simulink model "simulation_w_switch_sln3"  (Simulink 10.1)
settings: Solver=VariableStepAuto  StartTime=0.0  StopTime=tTot  MaxStep=1e-5  RelTol=1e-5
PreLoadFcn:
  | syst_init
values from neighbouring files (symbols this model uses):
  Aij = Aconn-Aii    [syst_init.m]
  AL = blkdiag(DGU.ALi)    [syst_init.m]
  atk24 = [zeros(3,1); 0.1*rand(3,1)-0.05]    [syst_init.m]
  atk34 = [zeros(3,1); 0.1*rand(3,1)-0.05]    [syst_init.m]
  B = blkdiag(DGU.B)    [syst_init.m]
  bC = blkdiag(DGU.bC)    [syst_init.m]
  bF = blkdiag(DGU.bF)    [syst_init.m]
  bH = blkdiag(DGU.bH)    [syst_init.m]
  bigCyComm = [zeros(3,3)  eye(3) zeros(3,30) ... (first row only)    [syst_init.m]
  bKhat = blkdiag(DGU.bKhat)    [syst_init.m]
  DGU = stateDyn(DGU,6)    [syst_init.m]
  F = blkdiag(DGU.Fj)    [syst_init.m]
  H = blkdiag(DGU.Hj)    [syst_init.m]
  K = blkdiag(DGU.K)    [syst_init.m]
  Khat = blkdiag(DGU.Khat)    [syst_init.m]
  L = blkdiag(DGU.Li)    [syst_init.m]
  n = 3    [syst_init.m]
  N = 6    [syst_init.m]
  nMaxMeas = .01    (= 0.01)    [syst_init.m]
  rhoMax = nMaxMeas*repmat([ones(n-1,1);0],N,1)    [syst_init.m]
  T = blkdiag(DGU.Tj)    [syst_init.m]
  Ta = 8    [syst_init.m]
  Tc = 2    [syst_init.m]
  tSampData = 1e-3    (= 0.001)    [syst_init.m]
  Vs = 60    [syst_init.m]
  wMax = nMax*repmat([ones(n-1,1);0],N,1)+nMaxMeas*repmat([zeros(n-1,1);1],N,1)    [syst_init.m]
undefined symbols (not defined in the file or in its folder): epsilon0bar, integral_Loc, rLoc_bar
libraries: powerlib x136, powerlib_meascontrol x13
(part 1 of 4)
settings Model: Creator=mustafa  LastModifiedBy=mustafa
settings DataIOCC: SaveFormat=Dataset
settings OptimizationCC: LifeSpan=auto
settings DebuggingCC: UnderspecifiedInitializationDetection=Simplified  MergeDetectMultiDrivingBlocksExec=error  UnconnectedInputMsg=none  UnconnectedOutputMsg=none  UnconnectedLineMsg=none  SFUnexpectedBacktrackingDiag=error  SFNoUnconditionalDefaultTransitionDiag=error  SFExecutionAtInitializationDiag=warning
settings HardwareCC: ProdBitPerPointer=64  ProdBitPerSizeT=64  ProdBitPerPtrDiffT=64  ProdLargestAtomicFloat=Float  ProdIntDivRoundTo=Zero  ProdEndianess=LittleEndian  ProdWordSize=64  ProdHWDeviceType=Intel->x86-64 (Windows64)
settings ModelReferenceCC: PropagateSignalLabelsOutOfModel=on
settings SFSimCC: SimUseLocalCustomCode=on
settings RTWCC: RTWUseLocalCustomCode=on
settings CodeAppCC: StateflowObjectComments=off
settings GRTTargetCC: TargetLangStandard=C99 (ISO)  CombineOutputUpdateFcns=on  GRTInterface=off
settings ConfigComp: CovMetricSettings=dwe  CovHtmlReporting=off  CovSaveCumulativeToWorkspaceVar=off  CovSaveSingleToWorkspaceVar=off  CovExternalEMLEnable=on

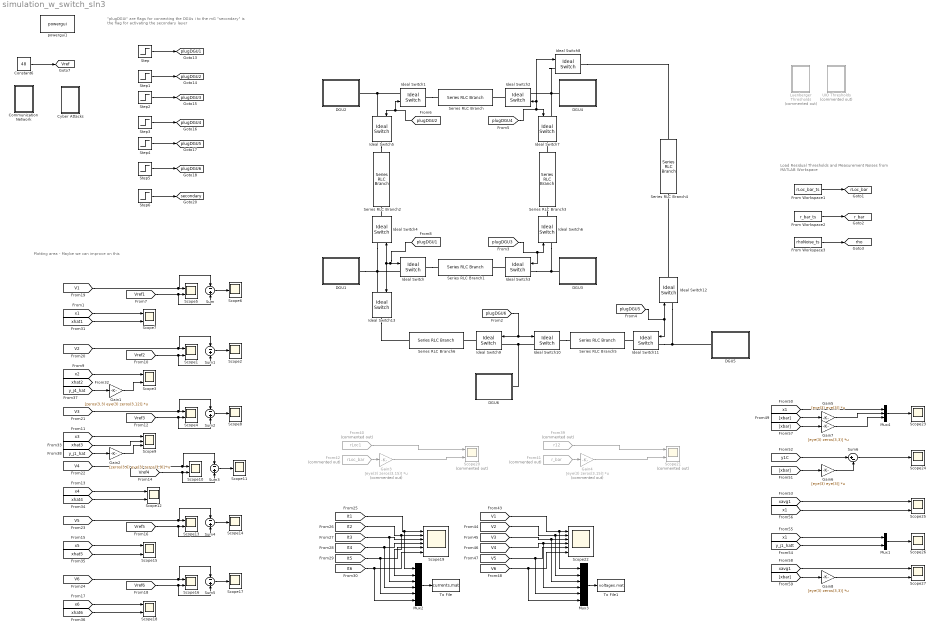
== system simulation_w_switch_sln3 ==
  note: Plotting area - Maybe we can improve on this
  note: "plugDGUi" are flags for connecting the DGUs i to the mG
      | "secondary" is the flag for activating the secondary layer
  note: Load Residual Thresholds and Measurement
      | Noises from MATLAB Workspace
  Communication  Network : Subsystem
  Constant6 : Constant  Value=48
  Cyber Attacks : Subsystem
  DGU1 : Subsystem
  DGU2 : Subsystem
  DGU3 : Subsystem
  DGU4 : Subsystem
  DGU5 : Subsystem
  DGU6 : Subsystem
  From Workspace1 : FromWorkspace  VariableName=rLoc_bar_ts
  From Workspace2 : FromWorkspace  VariableName=r_bar_ts
  From Workspace3 : FromWorkspace  VariableName=rhoNoise_ts
  From39 : From  Commented=on  GotoTag=r12  TagVisibility=global
  From40 : From  Commented=on  GotoTag=rLoc1  TagVisibility=global
  From41 : From  Commented=on  GotoTag=r_bar  TagVisibility=global
  From42 : From  Commented=on  GotoTag=rLoc_bar  TagVisibility=global
  Gain1 : Gain  Gain=[zeros(3,3) eye(3) zeros(3,12)]  Multiplication=Matrix(K*u) (u vector)
  Gain2 : Gain  Gain=[zeros(3,6) eye(3) zeros(3,9)]  Multiplication=Matrix(K*u) (u vector)
  Gain3 : Gain  Commented=on  Gain=[eye(3) zeros(3,15)]  Multiplication=Matrix(K*u) (u vector)
  Gain4 : Gain  Commented=on  Gain=[eye(3) zeros(3,15)]  Multiplication=Matrix(K*u) (u vector)
  Gain5 : Gain  Gain=[eye(3) eye(3)]  Multiplication=Matrix(K*u) (u vector)
  Gain6 : Gain  Gain=[eye(3) eye(3)]  Multiplication=Matrix(K*u) (u vector)
  Gain7 : Gain  Gain=[eye(3) zeros(3,3)]  Multiplication=Matrix(K*u) (u vector)
  Gain8 : Gain  Gain=[eye(3) zeros(3,3)]  Multiplication=Matrix(K*u) (u vector)
  Ideal Switch{,1..13} (14 alike) : powerlib/Power Electronics/Ideal Switch  Ron=0.001  Lon=0  IC=0  Rs=1e5  Cs=inf  Measurements=off
  Luenberger Thresholds : Subsystem  Commented=on
  Mux1 : Mux  Inputs=2
  Mux2 : Mux  Inputs=6
  Mux3 : Mux  Inputs=6
  Mux4 : Mux  Inputs=3
  Scope{1,4..5,7,10,12..13,15..16,18,25,27} (12 alike) : Scope  NumInputPorts=2
  Scope{2,6,8,11,14,17,23..24,26} (9 alike) : Scope
  Scope19 : Scope  NumInputPorts=6
  Scope20 : Scope  Commented=on  NumInputPorts=2
  Scope21 : Scope  Commented=on  NumInputPorts=2
  Scope22 : Scope  NumInputPorts=6
  Scope3 : Scope  NumInputPorts=3
  Scope9 : Scope  NumInputPorts=3
  Series RLC Branch : powerlib/Elements/Series RLC Branch  LConnTagsString=__new0  RConnTagsString=__new0  BranchType=RL  Resistance=DGU(2).Rij(2)  Inductance=DGU(2).Lij(2)  SetiL0=off  InitialCurrent=0  Capacitance=1e-6  Setx0=off  InitialVoltage=0  Measurements=None
  Series RLC Branch1 : powerlib/Elements/Series RLC Branch  LConnTagsString=__new0  RConnTagsString=__new0  BranchType=RL  Resistance=DGU(1).Rij(2)  Inductance=DGU(1).Lij(2)  SetiL0=off  InitialCurrent=0  Capacitance=1e-6  Setx0=off  InitialVoltage=0  Measurements=None
  Series RLC Branch2 : powerlib/Elements/Series RLC Branch  LConnTagsString=__new0  RConnTagsString=__new0  BranchType=RL  Resistance=DGU(1).Rij(1)  Inductance=DGU(1).Lij(1)  SetiL0=off  InitialCurrent=0  Capacitance=1e-6  Setx0=off  InitialVoltage=0  Measurements=None
  Series RLC Branch3 : powerlib/Elements/Series RLC Branch  LConnTagsString=__new0  RConnTagsString=__new0  BranchType=RL  Resistance=DGU(3).Rij(2)  Inductance=DGU(3).Lij(2)  SetiL0=off  InitialCurrent=0  Capacitance=1e-6  Setx0=off  InitialVoltage=0  Measurements=None
  Series RLC Branch4 : powerlib/Elements/Series RLC Branch  LConnTagsString=__new0  RConnTagsString=__new0  BranchType=RL  Resistance=DGU(4).Rij(3)  Inductance=DGU(4).Lij(3)  SetiL0=off  InitialCurrent=0  Capacitance=1e-6  Setx0=off  InitialVoltage=0  Measurements=None
  Series RLC Branch5 : powerlib/Elements/Series RLC Branch  LConnTagsString=__new0  RConnTagsString=__new0  BranchType=RL  Resistance=DGU(5).Rij(2)  Inductance=DGU(5).Lij(2)  SetiL0=off  InitialCurrent=0  Capacitance=1e-6  Setx0=off  InitialVoltage=0  Measurements=None
  Series RLC Branch6 : powerlib/Elements/Series RLC Branch  LConnTagsString=__new0  RConnTagsString=__new0  BranchType=RL  Resistance=DGU(1).Rij(3)  Inductance=DGU(1).Lij(3)  SetiL0=off  InitialCurrent=0  Capacitance=1e-6  Setx0=off  InitialVoltage=0  Measurements=None
  Step{,1..6} (7 alike) : Step  Time=Tc  SampleTime=0
  Sum{,1..5} (6 alike) : Sum  Inputs=-|+
  Sum6 : Sum  Inputs=|+-
  To File : ToFile  Filename=currents.mat  MatrixName=currents  SaveFormat=Timeseries  SampleTime=tSampData
  To File1 : ToFile  Filename=voltages.mat  MatrixName=voltages  SaveFormat=Timeseries  SampleTime=tSampData
  UIO Thresholds : Subsystem  Commented=on
  powergui1 : powerlib/powergui  Priority=1  SimulationMode=Continuous  SampleTime=50e-6  frequency=60  Iterations=50  frequencyindice=0  Pbase=100e6  ErrMax=1e-4  UnitsV=kV  UnitsW=MW  buscounter=0  FunctionMessages=off  echomessages=off  EnableUseOfTLC=off  CurrentSourceSwitches=off  DisableSnubberDevices=off  DisableRonSwitches=off  DisableVfSwitches=off  DisplayEquations=off  AutomaticDiscreteSolvers=off  SolverType=Tustin/Backward Euler (TBE)  Interpol=off  ExternalGateDelay=off  methode=off  Ts=100  x0status=blocks  SPID=on  SwTol=0  HookPort=off  NonlinearTolerance=1e-4  nMaxIteration=100  ContinueOnMaxIteration=off  RestoreLinks=warning  ResistiveCurrentMeasurement=off  Frange=[0:2:500]  Ylog=off  Xlog=on  ShowGrid=off  save=off  variable=ZData  structure=0  ZoomFFT=off  StartTime=0.0  cycles=1  DisplayStyle=1  fundamental=60  FreqAxis=off  MaxFrequency=1000  frequencyindicesteady=1  RmsSteady=1  display=off
  tag scope: Vref=global, plugDGU1=global, plugDGU2=global, plugDGU3=global, plugDGU4=global, plugDGU5=global, plugDGU6=global, rLoc_bar=global, r_bar=global, rho=global, secondary=global
  wires:
  [Vref1] -> Sum/2, Scope5/2
  [V1] -> Sum/1, Scope5/1
  Sum/1 -> Scope6/1
  [x1] -> Scope7/1
  [plugDGU2] -> Ideal Switch1/1, Ideal Switch5/1
  [plugDGU1] -> Ideal Switch4/1, Ideal Switch13/1, Ideal Switch/1
  [plugDGU3] -> Ideal Switch6/1, Ideal Switch3/1
  [plugDGU4] -> Ideal Switch7/1, Ideal Switch8/1, Ideal Switch2/1
  [plugDGU6] -> Ideal Switch9/1, Ideal Switch10/1
  [plugDGU5] -> Ideal Switch11/1, Ideal Switch12/1
  [V2] -> Sum1/1, Scope1/1
  [Vref2] -> Sum1/2, Scope1/2
  Sum1/1 -> Scope2/1
  [x2] -> Scope3/1
  [V3] -> Sum2/1, Scope4/1
  [Vref3] -> Sum2/2, Scope4/2
  Sum2/1 -> Scope8/1
  [x3] -> Scope9/1
  [V4] -> Sum3/1, Scope10/1
  [Vref4] -> Sum3/2, Scope10/2
  Sum3/1 -> Scope11/1
  [x4] -> Scope12/1
  [V5] -> Sum4/1, Scope13/1
  [Vref5] -> Sum4/2, Scope13/2
  Sum4/1 -> Scope14/1
  [x5] -> Scope15/1
  [V6] -> Sum5/1, Scope16/1
  [Vref6] -> Sum5/2, Scope16/2
  Sum5/1 -> Scope17/1
  [x6] -> Scope18/1
  Step/1 -> [plugDGU1]
  Step1/1 -> [plugDGU2]
  Step2/1 -> [plugDGU3]
  Step3/1 -> [plugDGU4]
  Step4/1 -> [plugDGU5]
  Step5/1 -> [plugDGU6]
  Constant6/1 -> [Vref]
  Step6/1 -> [secondary]
  [It3] -> Mux2/3, Scope19/3
  [It2] -> Mux2/2, Scope19/2
  [It1] -> Mux2/1, Scope19/1
  [It4] -> Mux2/4, Scope19/4
  [It5] -> Mux2/5, Scope19/5
  [It6] -> Mux2/6, Scope19/6
  [xhat1] -> Scope7/2
  [xhat3] -> Scope9/2
  [xhat4] -> Scope12/2
  [xhat5] -> Scope15/2
  [xhat6] -> Scope18/2
  [y_j4_hat] -> Gain1/1
  Gain1/1 -> Scope3/3
  [y_j1_hat] -> Gain2/1
  Gain2/1 -> Scope9/3
  From42/1 -> Gain3/1
  From41/1 -> Gain4/1
  From40/1 -> Scope20/1
  Gain4/1 -> Scope21/2
  Gain3/1 -> Scope20/2
  From39/1 -> Scope21/1
  [V6] -> Mux3/6, Scope22/6
  [V1] -> Mux3/1, Scope22/1
  [V4] -> Scope22/4, Mux3/4
  [V3] -> Mux3/3, Scope22/3
  [V2] -> Mux3/2, Scope22/2
  [V5] -> Mux3/5, Scope22/5
  Mux4/1 -> Scope23/1
  [x1] -> Mux4/1
  Sum6/1 -> Scope24/1
  Gain5/1 -> Mux4/2
  [xbar] -> Gain6/1
  Gain6/1 -> Sum6/2
  [xbar] -> Gain5/1
  [y1C] -> Sum6/1
  [xavg1] -> Scope25/1
  [y_j1_hatt] -> Mux1/2
  [x1] -> Mux1/1
  Mux1/1 -> Scope26/1
  [x1] -> Scope25/2
  [xbar] -> Gain7/1
  Gain7/1 -> Mux4/3
  [xavg1] -> Scope27/1
  [xbar] -> Gain8/1
  Gain8/1 -> Scope27/2
  From Workspace1/1 -> [rLoc_bar]
  From Workspace2/1 -> [r_bar]
  From Workspace3/1 -> [rho]
  Mux2/1 -> To File/1
  Mux3/1 -> To File1/1
  connections:
  Ideal Switch/RConn1 -- Series RLC Branch1/LConn1
  Ideal Switch1/RConn1 -- Series RLC Branch/LConn1
  Ideal Switch4/RConn1 -- Series RLC Branch2/RConn1
  DGU1/RConn1 -- Ideal Switch13/LConn1 -- Ideal Switch4/LConn1 -- Ideal Switch/LConn1
  Ideal Switch5/RConn1 -- Series RLC Branch2/LConn1
  Ideal Switch1/LConn1 -- Ideal Switch5/LConn1 -- DGU2/RConn1
  Ideal Switch3/RConn1 -- Series RLC Branch1/RConn1
  Ideal Switch2/RConn1 -- Series RLC Branch/RConn1
  Ideal Switch3/LConn1 -- Ideal Switch6/LConn1 -- DGU3/LConn1
  Ideal Switch2/LConn1 -- Ideal Switch8/LConn1 -- Ideal Switch7/LConn1 -- DGU4/LConn1
  Series RLC Branch3/LConn1 -- Ideal Switch7/RConn1
  Series RLC Branch3/RConn1 -- Ideal Switch6/RConn1
  Ideal Switch8/RConn1 -- Series RLC Branch4/LConn1
  Ideal Switch9/RConn1 -- Series RLC Branch6/RConn1
  Ideal Switch10/RConn1 -- Series RLC Branch5/LConn1
  Ideal Switch10/LConn1 -- Ideal Switch9/LConn1 -- DGU6/RConn1
  Ideal Switch11/RConn1 -- Series RLC Branch5/RConn1
  Ideal Switch11/LConn1 -- Ideal Switch12/LConn1 -- DGU5/LConn1
  Ideal Switch13/RConn1 -- Series RLC Branch6/LConn1
  Ideal Switch12/RConn1 -- Series RLC Branch4/RConn1

== system simulation_w_switch_sln3/Communication  Network ==
  Constant : Constant  Value=zeros(2*n*N,1)
  Gain : Gain  Gain=blkdiag(zeros(6),eye(6),eye(6),zeros(6),zeros(6),eye(6))  Multiplication=Matrix(K*u) (u vector)
  Gain1 : Gain  Gain=blkdiag(eye(6),zeros(6),zeros(6),eye(6),zeros(6),zeros(6))  Multiplication=Matrix(K*u) (u vector)
  Gain2 : Gain  Gain=blkdiag(eye(6),zeros(6),zeros(6),eye(6),zeros(6),zeros(6))  Multiplication=Matrix(K*u) (u vector)
  Gain3 : Gain  Gain=blkdiag(zeros(6),eye(6),eye(6),zeros(6),eye(6),zeros(6))  Multiplication=Matrix(K*u) (u vector)
  Gain4 : Gain  Gain=blkdiag(zeros(6),zeros(6),zeros(6),eye(6),zeros(6),eye(6))  Multiplication=Matrix(K*u) (u vector)
  Gain5 : Gain  Gain=blkdiag(eye(6),zeros(6),zeros(6),zeros(6),eye(6),zeros(6))  Multiplication=Matrix(K*u) (u vector)
  Mux : Mux  Inputs=12
  Switch : Switch  Criteria=u2 > Threshold  Threshold=0.1
  tag scope: yCom1=global, yCom2=global, yCom3=global, yCom4=global, yCom5=global, yCom6=global, yTot=global
  wires:
  [y1] -> Mux/2
  Gain/1 -> [yCom1]
  Gain3/1 -> [yCom4]
  [y6] -> Mux/12
  [y5] -> Mux/10
  [y4] -> Mux/8
  [yTot] -> Gain1/1, Gain2/1, Gain3/1, Gain4/1, Gain5/1, Gain/1
  Gain5/1 -> [yCom6]
  [y3] -> Mux/6
  [y2] -> Mux/4
  Gain4/1 -> [yCom5]
  Gain1/1 -> [yCom2]
  Gain2/1 -> [yCom3]
  Constant/1 -> Switch/3
  [secondary] -> Switch/2
  Switch/1 -> [yTot]
  Mux/1 -> Switch/1
  [xavg6] -> Mux/11
  [xavg1] -> Mux/1
  [xavg2] -> Mux/3
  [xavg3] -> Mux/5
  [xavg4] -> Mux/7
  [xavg5] -> Mux/9

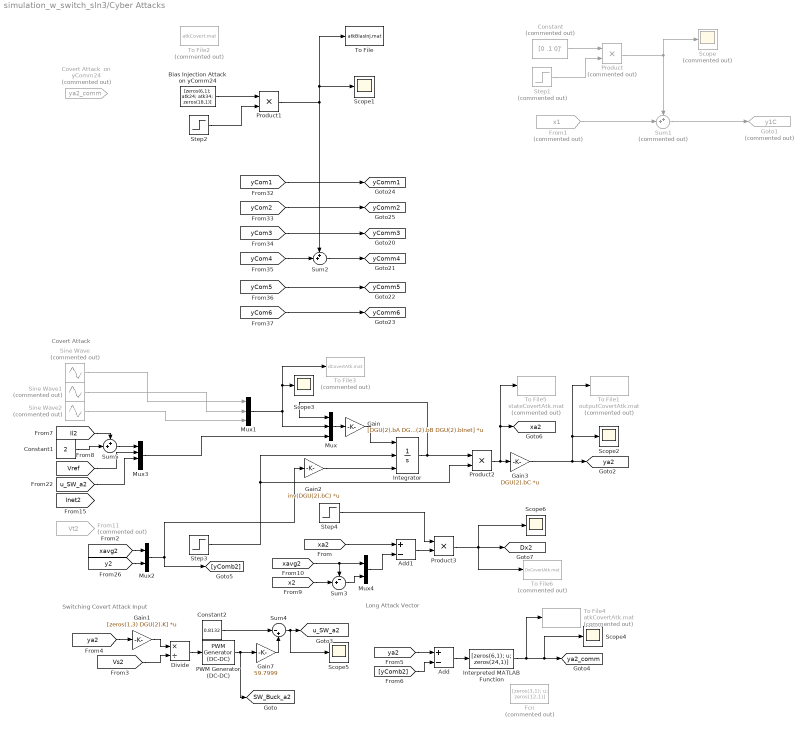
== system simulation_w_switch_sln3/Cyber Attacks ==
  note: Long Attack Vector
  note: Switching Covert Attack Input
  note: Covert Attack
  Add : Sum  Inputs=+-
  Add1 : Sum  Inputs=+-
  Bias Injection Attack on yComm24 : Constant  Value=[zeros(6,1); atk24; atk34; zeros(18,1)]
  Constant : Constant  Commented=on  Value=[0 .1 0]'
  Constant1 : Constant  Value=2
  Constant2 : Constant  Value=0.8132
  Covert Attack  on yComm24 : From  Commented=on  GotoTag=ya2_comm  TagVisibility=global
  Divide : Product  Inputs=*/
  Fcn : Fcn  Commented=on  Expr=[zeros(3,1); u; zeros(12,1)]
  From1 : From  Commented=on  GotoTag=x1  TagVisibility=global
  From11 : From  Commented=on  GotoTag=Vt2  TagVisibility=global
  Gain : Gain  Gain=[DGU(2).bA DGU(2).bEbar DGU(2).bM DGU(2).bB DGU(2).bInet]  Multiplication=Matrix(K*u) (u vector)
  Gain1 : Gain  Gain=[zeros(1,3) DGU(2).K]  Multiplication=Matrix(K*u) (u vector)
  Gain2 : Gain  Gain=inv(DGU(2).bC)  Multiplication=Matrix(K*u) (u vector)
  Gain3 : Gain  Gain=DGU(2).bC  Multiplication=Matrix(K*u) (u vector)
  Gain7 : Gain  Gain=59.7999
  Goto1 : Goto  Commented=on  GotoTag=y1C  TagVisibility=global
  Integrator : Integrator  ExternalReset=rising  InitialConditionSource=external
  Interpreted MATLAB Function : MATLABFcn  MATLABFcn=[zeros(6,1); u; zeros(24,1)]
  Mux : Mux  Inputs=3
  Mux1 : Mux  Inputs=3
  Mux2 : Mux  Inputs=2
  Mux3 : Mux
  Mux4 : Mux  Inputs=2
  PWM Generator (DC-DC) : powerlib_meascontrol/Pulse & Signal Generators/PWM Generator (DC-DC)  Fsw=10000  Ts=0
  Product : Product  Commented=on
  Product1 : Product
  Product2 : Product
  Product3 : Product
  Scope : Scope  Commented=on
  Scope{1..6} (6 alike) : Scope
  Sine Wave : Sin  Commented=on  Amplitude=1.2  Bias=1  Frequency=2*pi*0.1  Phase=90  SampleTime=0
  Sine Wave1 : Sin  Commented=on  Bias=0.5  Frequency=2*pi*0.2  SampleTime=0
  Sine Wave2 : Sin  Commented=on  Amplitude=0.8  Bias=0.6  Frequency=2*pi*0.15  SampleTime=0
  Step1 : Step  Commented=on  Time=8  SampleTime=0
  Step2 : Step  Time=Ta  SampleTime=0
  Step3 : Step  Time=Ta  SampleTime=0
  Step4 : Step  Time=Ta  SampleTime=0
  Sum1 : Sum  Commented=on  Inputs=++|
  Sum2 : Sum  Inputs=++|
  Sum3 : Sum  Inputs=-+|
  Sum4 : Sum  Inputs=|-+
  Sum5 : Sum  Inputs=++|
  To File : ToFile  Filename=atkBiasInj.mat  MatrixName=atkBiasInj  SaveFormat=Timeseries  SampleTime=tSampData
  To File1 : ToFile  Commented=on  Filename=outputCovertAtk.mat  MatrixName=outputCovertAtk  SaveFormat=Timeseries  SampleTime=tSampData
  To File2 : ToFile  Commented=on  Filename=atkCovert.mat  MatrixName=atkCovert  SaveFormat=Timeseries  SampleTime=tSampData
  To File3 : ToFile  Commented=on  Filename=dCovertAtk.mat  MatrixName=dCovertAtk  SaveFormat=Timeseries  SampleTime=tSampData
  To File4 : ToFile  Commented=on  Filename=atkCovertAtk.mat  MatrixName=atkCovertAtk  SaveFormat=Timeseries  SampleTime=tSampData
  To File5 : ToFile  Commented=on  Filename=stateCovertAtk.mat  MatrixName=stateCovertAtk  SaveFormat=Timeseries  SampleTime=tSampData
  To File6 : ToFile  Commented=on  Filename=DxCovertAtk.mat  MatrixName=DxCovertAtk  SaveFormat=Timeseries  SampleTime=tSampData
  tag scope: Dx2=global, SW_Buck_a2=global, u_SW_a2=global, xa2=global, yComm1=global, yComm2=global, yComm3=global, yComm4=global, yComm5=global, yComm6=global, ya2=global, ya2_comm=global
  wires:
  [yCom1] -> [yComm1]
  [yCom2] -> [yComm2]
  [yCom4] -> Sum2/2
  [yCom5] -> [yComm5]
  [yCom6] -> [yComm6]
  [yCom3] -> [yComm3]
  From1/1 -> Sum1/2
  Sum1/1 -> Goto1/1
  Constant/1 -> Product/1
  Product/1 -> Scope/1, Sum1/1
  Step1/1 -> Product/2
  Step2/1 -> Product1/2
  Product1/1 -> Sum2/1, To File/1, Scope1/1
  Bias Injection Attack on yComm24/1 -> Product1/1
  Sum2/1 -> [yComm4]
  Integrator/1 -> Product2/1, Mux/1
  Step3/1 -> Integrator/2, Product2/2
  Gain/1 -> Integrator/1
  [Vs2] -> Divide/2
  Gain1/1 -> Divide/1
  Divide/1 -> PWM Generator (DC-DC)/1
  [ya2] -> Gain1/1
  Gain7/1 -> Sum4/2
  PWM Generator (DC-DC)/1 -> Gain7/1, [SW_Buck_a2]
  Constant2/1 -> Sum4/1
  Sum4/1 -> Scope5/1, [u_SW_a2]
  Mux/1 -> Gain/1
  Mux1/1 -> Scope3/1, To File3/1, Mux/2
  Sine Wave/1 -> Mux1/1
  Sine Wave1/1 -> Mux1/2
  Product2/1 -> To File5/1, [xa2], Gain3/1
  [ya2] -> Add/1
  [yComb2] -> Add/2
  Add/1 -> Interpreted MATLAB Function/1
  Interpreted MATLAB Function/1 -> To File4/1, Scope4/1, [ya2_comm]
  Mux2/1 -> [yComb2], Gain2/1
  Gain2/1 -> Integrator/3
  [xavg2] -> Mux2/1
  [y2] -> Mux2/2
  Sine Wave2/1 -> Mux1/3
  Gain3/1 -> To File1/1, Scope2/1, [ya2]
  [Il2] -> Sum5/1
  [Vref] -> Mux3/2
  [u_SW_a2] -> Mux3/3
  Mux3/1 -> Mux/3
  [xa2] -> Add1/1
  [xavg2] -> Sum3/1, Mux4/1
  Mux4/1 -> Add1/2
  [x2] -> Sum3/2
  Sum3/1 -> Mux4/2
  Constant1/1 -> Sum5/2
  Sum5/1 -> Mux3/1
  Add1/1 -> Product3/2
  Step4/1 -> Product3/1
  Product3/1 -> To File6/1, [Dx2], Scope6/1

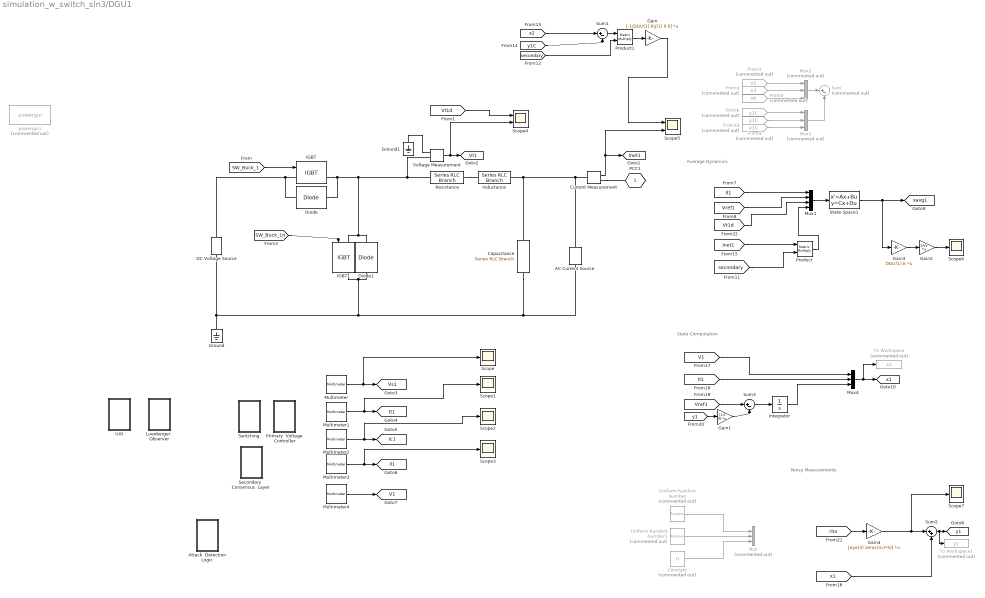
== system simulation_w_switch_sln3/DGU1 ==
  note: Average Dynamics
  note: Noisy Measurements
  note: State Computation
  AC Current Source : powerlib/Electrical Sources/AC Current Source  Amplitude=10  Phase=90  Frequency=0  SampleTime=0  Measurements=Current
      settings: SourceProductBaseCode=PS
  Attack  Detection Logic : Subsystem
  Capacitance : powerlib/Elements/Series RLC Branch  LConnTagsString=__new0  RConnTagsString=__new0  BranchType=C  Resistance=1  Inductance=1.8e-3  SetiL0=off  InitialCurrent=0  Capacitance=DGU(1).Ct  Setx0=off  InitialVoltage=48  Measurements=Branch voltage and current
  Constant : Constant  Commented=on  Value=0
  Current Measurement : powerlib/Measurements/Current Measurement  PhasorSimulation=off  OutputType=Magnitude  PSBequivalent=0
  DC Voltage Source : powerlib/Electrical Sources/DC Voltage Source  Amplitude=Vs  Measurements=Voltage
  Diode : powerlib/Power Electronics/Diode  Ron=0.001  Lon=0  Vf=0.8  IC=0  UseSnubber=0  Rs=500  Cs=250e-9  Measurements=off
  Diode1 : powerlib/Power Electronics/Diode  Ron=0.001  Lon=0  Vf=0.8  IC=0  UseSnubber=0  Rs=500  Cs=250e-9  Measurements=off
  From10 : From  Commented=on  GotoTag=y1C  TagVisibility=global
  From3 : From  Commented=on  GotoTag=x2  TagVisibility=global
  From4 : From  Commented=on  GotoTag=x3  TagVisibility=global
  From5 : From  Commented=on  GotoTag=x6  TagVisibility=global
  From6 : From  Commented=on  GotoTag=y1C  TagVisibility=global
  From9 : From  Commented=on  GotoTag=y1C  TagVisibility=global
  Gain : Gain  Gain=[-1/DGU(1).Rij(1) 0 0]  Multiplication=Matrix(K*u) (u vector)
  Gain1 : Gain  Gain=[1 0 0]  Multiplication=Matrix(K*u) (u vector)
  Gain2 : Gain  Gain=1/Vs  Multiplication=Matrix(K*u) (u vector)
  Gain3 : Gain  Gain=DGU(1).K  Multiplication=Matrix(K*u) (u vector)
  Gain4 : Gain  Gain=[eye(3) zeros(3,n*5)]  Multiplication=Matrix(K*u) (u vector)
  Ground : powerlib/Elements/Ground  LConnTagsString=a
  Ground1 : powerlib/Elements/Ground  LConnTagsString=a
  IGBT : powerlib/Power Electronics/IGBT  Ron=0.001  Lon=0  Vf=1  Tf=1e-6  Tt=2e-6  IC=0  Rs=1e5  Cs=inf  Measurements=on
  IGBT1 : powerlib/Power Electronics/IGBT  Ron=0.001  Lon=0  Vf=1  Tf=1e-6  Tt=2e-6  IC=0  Rs=1e5  Cs=inf  Measurements=on
  Inductance : powerlib/Elements/Series RLC Branch  LConnTagsString=__new0  RConnTagsString=__new0  BranchType=L  Resistance=1  Inductance=DGU(1).Lt  SetiL0=off  InitialCurrent=10  Capacitance=1e-6  Setx0=off  InitialVoltage=0  Measurements=None
  Integrator : Integrator
  Luenberger  Observer : Subsystem
  Multimeter : powerlib/Measurements/Multimeter  PhasorSimulation=off  OutputType=Complex  sel=7  L=30  Gain=1  yselected={'Usrc: DGU1/DC Voltage Source'};  PSBOutputType=1  PSBequivalent=0  AxesSetting=[0,0.1,-100,100]  Display=0  SavedBlockNames=-11
  Multimeter1 : powerlib/Measurements/Multimeter  PhasorSimulation=off  OutputType=Complex  sel=22  L=30  Gain=1  yselected={'Ib: DGU1/Resistance'};  PSBOutputType=1  PSBequivalent=0  AxesSetting=[0,0.1,-100,100]  Display=0  SavedBlockNames=-11
  Multimeter2 : powerlib/Measurements/Multimeter  PhasorSimulation=off  OutputType=Complex  sel=21  L=30  Gain=1  yselected={'Ib: DGU1/Capacitance'};  PSBOutputType=1  PSBequivalent=0  AxesSetting=[0,0.1,-100,100]  Display=0  SavedBlockNames=-11
  Multimeter3 : powerlib/Measurements/Multimeter  PhasorSimulation=off  OutputType=Complex  sel=25  L=30  Gain=1  yselected={'Isrc: DGU1/AC Current Source'};  PSBOutputType=1  PSBequivalent=0  AxesSetting=[0,0.1,-100,100]  Display=0  SavedBlockNames=-11
  Multimeter4 : powerlib/Measurements/Multimeter  PhasorSimulation=off  OutputType=Complex  sel=5  L=30  Gain=1  yselected={'Ub: DGU1/Capacitance'};  PSBOutputType=1  PSBequivalent=0  AxesSetting=[0,0.1,-100,100]  Display=0  SavedBlockNames=-11
  Mux : Mux  Commented=on  Inputs=3
  Mux1 : Mux
  Mux2 : Mux  Commented=on  Inputs=3
  Mux3 : Mux  Commented=on  Inputs=3
  Mux4 : Mux  Inputs=3
  Primary  Voltage  Controller : Subsystem
  Product : Product  Multiplication=Matrix(*)
  Product1 : Product  Multiplication=Matrix(*)
  Resistance : powerlib/Elements/Series RLC Branch  LConnTagsString=__new0  RConnTagsString=__new0  BranchType=R  Resistance=DGU(1).Rt  Inductance=1e-3  SetiL0=off  InitialCurrent=0  Capacitance=1e-6  Setx0=off  InitialVoltage=0  Measurements=Branch current
  Scope{,1..3,6..7} (6 alike) : Scope
  Scope4 : Scope  NumInputPorts=2
  Scope5 : Scope  NumInputPorts=2
  Secondary  Consensus  Layer : Subsystem
  State-Space1 : StateSpace  A=DGU(1).Aii  B=[DGU(1).M DGU(1).B [-1/DGU(1).Ct;0;0]]  C=eye(3)  D=zeros(n,4)  InitialCondition=0
  Sum : Sum  Commented=on  Inputs=|+-
  Sum1 : Sum  Inputs=|+-
  Sum2 : Sum  Inputs=|++
  Sum3 : Sum  Inputs=|+-
  Switching : Subsystem
  To Workspace : ToWorkspace  Commented=on  VariableName=x1  SaveFormat=Timeseries  SampleTime=tSampData
  To Workspace1 : ToWorkspace  Commented=on  VariableName=y1  SaveFormat=Timeseries  SampleTime=tSampData
  UIO : Subsystem
  Uniform Random Number : UniformRandomNumber  Commented=on  Minimum=-nMaxMeas  Maximum=nMaxMeas  Seed=1  SampleTime=0.1
  Uniform Random Number1 : UniformRandomNumber  Commented=on  Minimum=-nMaxMeas  Maximum=nMaxMeas  Seed=2  SampleTime=0.1
  Voltage Measurement : powerlib/Measurements/Voltage Measurement  PhasorSimulation=off  OutputType=Complex  PSBequivalent=0
  powergui1 : powerlib/powergui  Priority=1  Commented=on  SimulationMode=Continuous  SampleTime=50e-6  frequency=60  Iterations=50  frequencyindice=60  Pbase=100e6  ErrMax=1e-4  UnitsV=kV  UnitsW=MW  buscounter=0  FunctionMessages=off  echomessages=off  EnableUseOfTLC=off  CurrentSourceSwitches=off  DisableSnubberDevices=off  DisableRonSwitches=off  DisableVfSwitches=off  DisplayEquations=off  AutomaticDiscreteSolvers=off  SolverType=Tustin/Backward Euler (TBE)  Interpol=off  ExternalGateDelay=off  methode=off  Ts=100  x0status=blocks  SPID=on  SwTol=0  HookPort=off  NonlinearTolerance=1e-4  nMaxIteration=100  ContinueOnMaxIteration=off  RestoreLinks=warning  ResistiveCurrentMeasurement=off  Frange=[0:2:500]  Ylog=off  Xlog=on  ShowGrid=off  save=off  variable=ZData  structure=0  ZoomFFT=off  StartTime=0.0  cycles=1  DisplayStyle=1  fundamental=60  FreqAxis=off  MaxFrequency=1000  frequencyindicesteady=1  RmsSteady=1  display=off
  PCC1 : PMIOPort  Tag=PMCPort  Side=Right
  tag scope: Ic1=global, Il1=global, Inet1=global, It1=global, V1=global, Vs1=global, Vt1=global, x1=global, xavg1=global, y1=global
  wires:
  Multimeter/1 -> Scope/1, [Vs1]
  Multimeter2/1 -> Scope2/1, [Ic1]
  Voltage Measurement/1 -> Scope4/2, [Vt1]
  Multimeter1/1 -> Scope1/1, [It1]
  [SW_Buck_1n] -> IGBT1/1
  Multimeter3/1 -> Scope3/1, [Il1]
  [SW_Buck_1] -> IGBT/1
  Multimeter4/1 -> [V1]
  [Vt1d] -> Scope4/1
  [Il1] -> Mux1/1
  [Vref1] -> Mux1/2
  Gain2/1 -> Scope6/1
  Mux1/1 -> State-Space1/1
  State-Space1/1 -> Gain3/1, [xavg1]
  Gain3/1 -> Gain2/1
  From3/1 -> Mux2/1
  From5/1 -> Mux2/3
  From4/1 -> Mux2/2
  From9/1 -> Mux3/2
  From10/1 -> Mux3/3
  From6/1 -> Mux3/1
  Mux2/1 -> Sum/1
  Mux3/1 -> Sum/2
  [Inet1] -> Product/1
  Product/1 -> Mux1/4
  [secondary] -> Product/2
  Current Measurement/1 -> [Inet1], Scope5/2
  Gain/1 -> Scope5/1
  [y1C] -> Sum1/2
  Product1/1 -> Gain/1
  Sum1/1 -> Product1/1
  [x2] -> Sum1/1
  [secondary] -> Product1/2
  [rho] -> Gain4/1
  [Vref1] -> Sum3/1
  [x1] -> Sum2/2
  Uniform Random Number/1 -> Mux/1
  Sum2/1 -> To Workspace1/1, [y1]
  [It1] -> Mux4/2
  Uniform Random Number1/1 -> Mux/2
  Constant/1 -> Mux/3
  [V1] -> Mux4/1
  Integrator/1 -> Mux4/3
  Sum3/1 -> Integrator/1
  [y1] -> Gain1/1
  Gain1/1 -> Sum3/2
  Gain4/1 -> Sum2/1, Scope7/1
  Mux4/1 -> To Workspace/1, [x1]
  [Vt1d] -> Mux1/3
  connections:
  Ground1/LConn1 -- Voltage Measurement/LConn2
  IGBT1/RConn1 -- AC Current Source/RConn1 -- Capacitance/RConn1 -- Ground/LConn1 -- DC Voltage Source/LConn1 -- Diode1/LConn1
  Capacitance/LConn1 -- Current Measurement/LConn1 -- AC Current Source/LConn1 -- Inductance/RConn1
  IGBT1/LConn1 -- Resistance/LConn1 -- Voltage Measurement/LConn1 -- IGBT/RConn1 -- Diode/LConn1 -- Diode1/RConn1
  IGBT/LConn1 -- Diode/RConn1 -- DC Voltage Source/RConn1
  Resistance/RConn1 -- Inductance/LConn1
  Current Measurement/RConn1 -- PCC1/RConn1

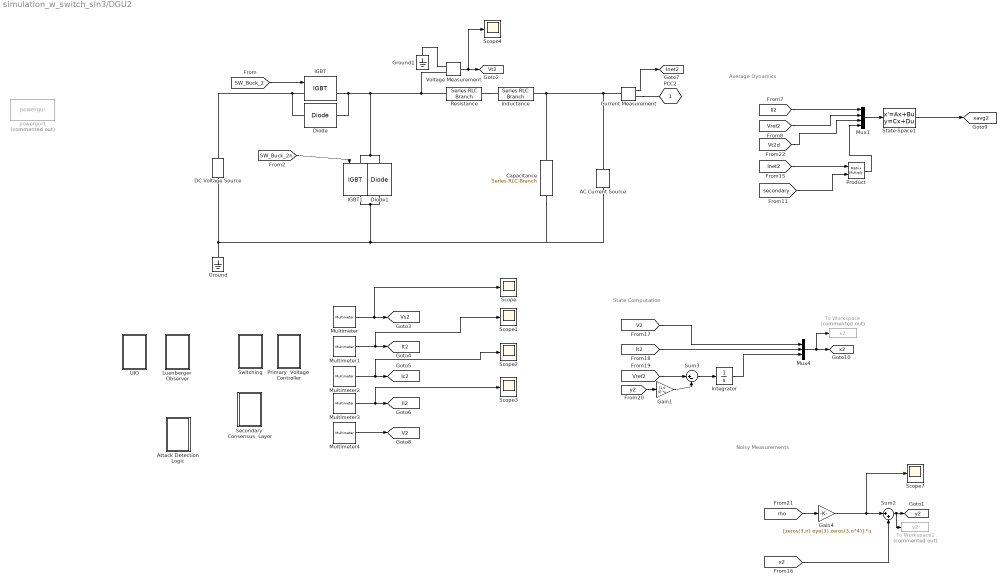
== system simulation_w_switch_sln3/DGU2 ==
  note: Noisy Measurements
  note: State Computation
  note: Average Dynamics
  AC Current Source : powerlib/Electrical Sources/AC Current Source  Amplitude=12  Phase=90  Frequency=0  SampleTime=0  Measurements=Current
      settings: SourceProductBaseCode=PS
  Attack Detection Logic : Subsystem
  Capacitance : powerlib/Elements/Series RLC Branch  LConnTagsString=__new0  RConnTagsString=__new0  BranchType=C  Resistance=1  Inductance=1.8e-3  SetiL0=off  InitialCurrent=0  Capacitance=DGU(2).Ct  Setx0=off  InitialVoltage=48  Measurements=Branch voltage and current
  Current Measurement : powerlib/Measurements/Current Measurement  PhasorSimulation=off  OutputType=Magnitude  PSBequivalent=0
  DC Voltage Source : powerlib/Electrical Sources/DC Voltage Source  Amplitude=Vs  Measurements=Voltage
  Diode : powerlib/Power Electronics/Diode  Ron=0.001  Lon=0  Vf=0.8  IC=0  UseSnubber=0  Rs=500  Cs=250e-9  Measurements=off
  Diode1 : powerlib/Power Electronics/Diode  Ron=0.001  Lon=0  Vf=0.8  IC=0  UseSnubber=0  Rs=500  Cs=250e-9  Measurements=off
  Gain1 : Gain  Gain=[1 0 0]  Multiplication=Matrix(K*u) (u vector)
  Gain4 : Gain  Gain=[zeros(3,n) eye(3) zeros(3,n*4)]  Multiplication=Matrix(K*u) (u vector)
  Ground : powerlib/Elements/Ground  LConnTagsString=a
  Ground1 : powerlib/Elements/Ground  LConnTagsString=a
  IGBT : powerlib/Power Electronics/IGBT  Ron=0.001  Lon=0  Vf=1  Tf=1e-6  Tt=2e-6  IC=0  Rs=1e5  Cs=inf  Measurements=on
  IGBT1 : powerlib/Power Electronics/IGBT  Ron=0.001  Lon=0  Vf=1  Tf=1e-6  Tt=2e-6  IC=0  Rs=1e5  Cs=inf  Measurements=on
  Inductance : powerlib/Elements/Series RLC Branch  LConnTagsString=__new0  RConnTagsString=__new0  BranchType=L  Resistance=1  Inductance=DGU(2).Lt  SetiL0=off  InitialCurrent=12  Capacitance=1e-6  Setx0=off  InitialVoltage=0  Measurements=None
  Integrator : Integrator
  Luenberger  Observer : Subsystem
  Multimeter : powerlib/Measurements/Multimeter  PhasorSimulation=off  OutputType=Complex  sel=8  L=30  Gain=1  yselected={'Usrc: DGU2/DC Voltage Source'};  PSBOutputType=1  PSBequivalent=0  AxesSetting=[0,0.1,-100,100]  Display=0  SavedBlockNames=-11
  Multimeter1 : powerlib/Measurements/Multimeter  PhasorSimulation=off  OutputType=Complex  sel=24  L=30  Gain=1  yselected={'Ib: DGU2/Resistance'};  PSBOutputType=1  PSBequivalent=0  AxesSetting=[0,0.1,-100,100]  Display=0  SavedBlockNames=-11
  Multimeter2 : powerlib/Measurements/Multimeter  PhasorSimulation=off  OutputType=Complex  sel=23  L=30  Gain=1  yselected={'Ib: DGU2/Capacitance'};  PSBOutputType=1  PSBequivalent=0  AxesSetting=[0,0.1,-100,100]  Display=0  SavedBlockNames=-11
  Multimeter3 : powerlib/Measurements/Multimeter  PhasorSimulation=off  OutputType=Complex  sel=26  L=30  Gain=1  yselected={'Isrc: DGU2/AC Current Source'};  PSBOutputType=1  PSBequivalent=0  AxesSetting=[0,0.1,-100,100]  Display=0  SavedBlockNames=-11
  Multimeter4 : powerlib/Measurements/Multimeter  PhasorSimulation=off  OutputType=Complex  sel=6  L=30  Gain=1  yselected={'Ub: DGU2/Capacitance'};  PSBOutputType=1  PSBequivalent=0  AxesSetting=[0,0.1,-100,100]  Display=0  SavedBlockNames=-11
  Mux1 : Mux
  Mux4 : Mux  Inputs=3
  Primary  Voltage  Controller : Subsystem
  Product : Product  Multiplication=Matrix(*)
  Resistance : powerlib/Elements/Series RLC Branch  LConnTagsString=__new0  RConnTagsString=__new0  BranchType=R  Resistance=DGU(2).Rt  Inductance=1e-3  SetiL0=off  InitialCurrent=0  Capacitance=1e-6  Setx0=off  InitialVoltage=0  Measurements=Branch current
  Scope{,1..4,7} (6 alike) : Scope
  Secondary  Consensus  Layer : Subsystem
  State-Space1 : StateSpace  A=DGU(2).Aii  B=[DGU(2).M DGU(2).B [-1/DGU(2).Ct;0;0]]  C=eye(3)  D=zeros(n,4)  InitialCondition=0
  Sum2 : Sum  Inputs=|++
  Sum3 : Sum  Inputs=|+-
  Switching : Subsystem
  To Workspace : ToWorkspace  Commented=on  VariableName=x2  SaveFormat=Timeseries  SampleTime=tSampData
  To Workspace1 : ToWorkspace  Commented=on  VariableName=y2  SaveFormat=Timeseries  SampleTime=tSampData
  UIO : Subsystem
  Voltage Measurement : powerlib/Measurements/Voltage Measurement  PhasorSimulation=off  OutputType=Complex  PSBequivalent=0
  powergui1 : powerlib/powergui  Priority=1  Commented=on  SimulationMode=Continuous  SampleTime=50e-6  frequency=60  Iterations=50  frequencyindice=60  Pbase=100e6  ErrMax=1e-4  UnitsV=kV  UnitsW=MW  buscounter=0  FunctionMessages=off  echomessages=off  EnableUseOfTLC=off  CurrentSourceSwitches=off  DisableSnubberDevices=off  DisableRonSwitches=off  DisableVfSwitches=off  DisplayEquations=off  AutomaticDiscreteSolvers=off  SolverType=Tustin/Backward Euler (TBE)  Interpol=off  ExternalGateDelay=off  methode=off  Ts=100  x0status=blocks  SPID=on  SwTol=0  HookPort=off  NonlinearTolerance=1e-4  nMaxIteration=100  ContinueOnMaxIteration=off  RestoreLinks=warning  ResistiveCurrentMeasurement=off  Frange=[0:2:500]  Ylog=off  Xlog=on  ShowGrid=off  save=off  variable=ZData  structure=0  ZoomFFT=off  StartTime=0.0  cycles=1  DisplayStyle=1  fundamental=60  FreqAxis=off  MaxFrequency=1000  frequencyindicesteady=1  RmsSteady=1  display=off
  PCC2 : PMIOPort  Tag=PMCPort  Side=Right
  tag scope: Ic2=global, Il2=global, Inet2=global, It2=global, V2=global, Vs2=global, Vt2=global, x2=global, xavg2=global, y2=global
  wires:
  Multimeter/1 -> Scope/1, [Vs2]
  Multimeter2/1 -> Scope2/1, [Ic2]
  Voltage Measurement/1 -> Scope4/1, [Vt2]
  Multimeter1/1 -> Scope1/1, [It2]
  [SW_Buck_2n] -> IGBT1/1
  Multimeter3/1 -> Scope3/1, [Il2]
  [SW_Buck_2] -> IGBT/1
  Multimeter4/1 -> [V2]
  [rho] -> Gain4/1
  Gain1/1 -> Sum3/2
  [V2] -> Mux4/1
  [Vref2] -> Sum3/1
  [y2] -> Gain1/1
  [It2] -> Mux4/2
  Gain4/1 -> Sum2/1, Scope7/1
  Integrator/1 -> Mux4/3
  Sum3/1 -> Integrator/1
  Sum2/1 -> To Workspace1/1, [y2]
  Mux4/1 -> To Workspace/1, [x2]
  [x2] -> Sum2/2
  [Il2] -> Mux1/1
  Current Measurement/1 -> [Inet2]
  Mux1/1 -> State-Space1/1
  Product/1 -> Mux1/4
  [Inet2] -> Product/1
  [Vref2] -> Mux1/2
  [secondary] -> Product/2
  [Vt2d] -> Mux1/3
  State-Space1/1 -> [xavg2]
  connections:
  Ground1/LConn1 -- Voltage Measurement/LConn2
  IGBT1/RConn1 -- AC Current Source/RConn1 -- Capacitance/RConn1 -- Ground/LConn1 -- DC Voltage Source/LConn1 -- Diode1/LConn1
  Capacitance/LConn1 -- Current Measurement/LConn1 -- AC Current Source/LConn1 -- Inductance/RConn1
  Diode/LConn1 -- IGBT/RConn1 -- Resistance/LConn1 -- Voltage Measurement/LConn1 -- IGBT1/LConn1 -- Diode1/RConn1
  IGBT/LConn1 -- Diode/RConn1 -- DC Voltage Source/RConn1
  Resistance/RConn1 -- Inductance/LConn1
  Current Measurement/RConn1 -- PCC2/RConn1

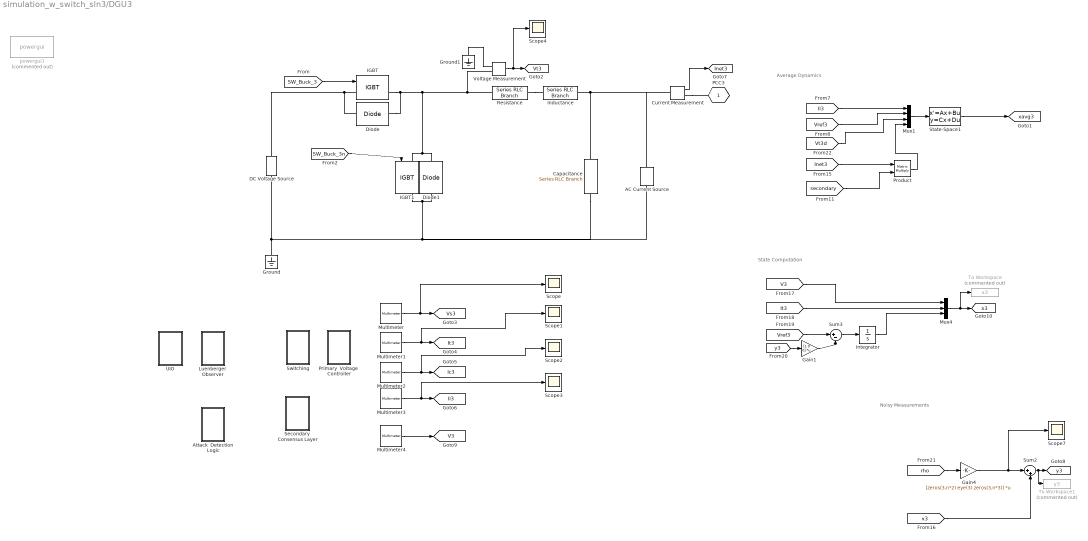
== system simulation_w_switch_sln3/DGU3 ==
  note: Noisy Measurements
  note: State Computation
  note: Average Dynamics
  AC Current Source : powerlib/Electrical Sources/AC Current Source  Amplitude=15  Phase=90  Frequency=0  SampleTime=0  Measurements=Current
      settings: SourceProductBaseCode=PS
  Attack  Detection Logic : Subsystem
  Capacitance : powerlib/Elements/Series RLC Branch  LConnTagsString=__new0  RConnTagsString=__new0  BranchType=C  Resistance=1  Inductance=1.8e-3  SetiL0=off  InitialCurrent=0  Capacitance=DGU(3).Ct  Setx0=off  InitialVoltage=48  Measurements=Branch voltage and current
  Current Measurement : powerlib/Measurements/Current Measurement  PhasorSimulation=off  OutputType=Magnitude  PSBequivalent=0
  DC Voltage Source : powerlib/Electrical Sources/DC Voltage Source  Amplitude=Vs  Measurements=Voltage
  Diode : powerlib/Power Electronics/Diode  Ron=0.001  Lon=0  Vf=0.8  IC=0  UseSnubber=0  Rs=500  Cs=250e-9  Measurements=off
  Diode1 : powerlib/Power Electronics/Diode  Ron=0.001  Lon=0  Vf=0.8  IC=0  UseSnubber=0  Rs=500  Cs=250e-9  Measurements=off
  Gain1 : Gain  Gain=[1 0 0]  Multiplication=Matrix(K*u) (u vector)
  Gain4 : Gain  Gain=[zeros(3,n*2) eye(3) zeros(3,n*3)]  Multiplication=Matrix(K*u) (u vector)
  Ground : powerlib/Elements/Ground  LConnTagsString=a
  Ground1 : powerlib/Elements/Ground  LConnTagsString=a
  IGBT : powerlib/Power Electronics/IGBT  Ron=0.001  Lon=0  Vf=1  Tf=1e-6  Tt=2e-6  IC=0  Rs=1e5  Cs=inf  Measurements=on
  IGBT1 : powerlib/Power Electronics/IGBT  Ron=0.001  Lon=0  Vf=1  Tf=1e-6  Tt=2e-6  IC=0  Rs=1e5  Cs=inf  Measurements=on
  Inductance : powerlib/Elements/Series RLC Branch  LConnTagsString=__new0  RConnTagsString=__new0  BranchType=L  Resistance=1  Inductance=DGU(3).Lt  SetiL0=off  InitialCurrent=15  Capacitance=1e-6  Setx0=off  InitialVoltage=0  Measurements=None
  Integrator : Integrator
  Luenberger  Observer : Subsystem
  Multimeter : powerlib/Measurements/Multimeter  PhasorSimulation=off  OutputType=Complex  sel=9  L=30  Gain=1  yselected={'Usrc: DGU3/DC Voltage Source'};  PSBOutputType=1  PSBequivalent=0  AxesSetting=[0,0.1,-100,100]  Display=0  SavedBlockNames=-11
  Multimeter1 : powerlib/Measurements/Multimeter  PhasorSimulation=off  OutputType=Complex  sel=14  L=30  Gain=1  yselected={'Ib: DGU3/Resistance'};  PSBOutputType=1  PSBequivalent=0  AxesSetting=[0,0.1,-100,100]  Display=0  SavedBlockNames=-11
  Multimeter2 : powerlib/Measurements/Multimeter  PhasorSimulation=off  OutputType=Complex  sel=13  L=30  Gain=1  yselected={'Ib: DGU3/Capacitance'};  PSBOutputType=1  PSBequivalent=0  AxesSetting=[0,0.1,-100,100]  Display=0  SavedBlockNames=-11
  Multimeter3 : powerlib/Measurements/Multimeter  PhasorSimulation=off  OutputType=Complex  sel=27  L=30  Gain=1  yselected={'Isrc: DGU3/AC Current Source'};  PSBOutputType=1  PSBequivalent=0  AxesSetting=[0,0.1,-100,100]  Display=0  SavedBlockNames=-11
  Multimeter4 : powerlib/Measurements/Multimeter  PhasorSimulation=off  OutputType=Complex  sel=1  L=30  Gain=1  yselected={'Ub: DGU3/Capacitance'};  PSBOutputType=1  PSBequivalent=0  AxesSetting=[0,0.1,-100,100]  Display=0  SavedBlockNames=-11
  Mux1 : Mux
  Mux4 : Mux  Inputs=3
  Primary  Voltage  Controller : Subsystem
  Product : Product  Multiplication=Matrix(*)
  Resistance : powerlib/Elements/Series RLC Branch  LConnTagsString=__new0  RConnTagsString=__new0  BranchType=R  Resistance=DGU(3).Rt  Inductance=1e-3  SetiL0=off  InitialCurrent=0  Capacitance=1e-6  Setx0=off  InitialVoltage=0  Measurements=Branch current
  Scope{,1..4,7} (6 alike) : Scope
  Secondary  Consensus Layer : Subsystem
  State-Space1 : StateSpace  A=DGU(3).Aii  B=[DGU(3).M DGU(3).B [-1/DGU(3).Ct;0;0]]  C=eye(3)  D=zeros(n,4)  InitialCondition=0
  Sum2 : Sum  Inputs=|++
  Sum3 : Sum  Inputs=|+-
  Switching : Subsystem
  To Workspace : ToWorkspace  Commented=on  VariableName=x3  SaveFormat=Timeseries  SampleTime=tSampData
  To Workspace1 : ToWorkspace  Commented=on  VariableName=y3  SaveFormat=Timeseries  SampleTime=tSampData
  UIO : Subsystem
  Voltage Measurement : powerlib/Measurements/Voltage Measurement  PhasorSimulation=off  OutputType=Complex  PSBequivalent=0
  powergui1 : powerlib/powergui  Priority=1  Commented=on  SimulationMode=Continuous  SampleTime=50e-6  frequency=60  Iterations=50  frequencyindice=60  Pbase=100e6  ErrMax=1e-4  UnitsV=kV  UnitsW=MW  buscounter=0  FunctionMessages=off  echomessages=off  EnableUseOfTLC=off  CurrentSourceSwitches=off  DisableSnubberDevices=off  DisableRonSwitches=off  DisableVfSwitches=off  DisplayEquations=off  AutomaticDiscreteSolvers=off  SolverType=Tustin/Backward Euler (TBE)  Interpol=off  ExternalGateDelay=off  methode=off  Ts=100  x0status=blocks  SPID=on  SwTol=0  HookPort=off  NonlinearTolerance=1e-4  nMaxIteration=100  ContinueOnMaxIteration=off  RestoreLinks=warning  ResistiveCurrentMeasurement=off  Frange=[0:2:500]  Ylog=off  Xlog=on  ShowGrid=off  save=off  variable=ZData  structure=0  ZoomFFT=off  StartTime=0.0  cycles=1  DisplayStyle=1  fundamental=60  FreqAxis=off  MaxFrequency=1000  frequencyindicesteady=1  RmsSteady=1  display=off
  PCC3 : PMIOPort  Tag=PMCPort  Side=Left
  tag scope: Ic3=global, Il3=global, Inet3=global, It3=global, V3=global, Vs3=global, Vt3=global, x3=global, xavg3=global, y3=global
  wires:
  Multimeter/1 -> Scope/1, [Vs3]
  Multimeter2/1 -> Scope2/1, [Ic3]
  Voltage Measurement/1 -> Scope4/1, [Vt3]
  Multimeter1/1 -> Scope1/1, [It3]
  [SW_Buck_3n] -> IGBT1/1
  Multimeter3/1 -> Scope3/1, [Il3]
  [SW_Buck_3] -> IGBT/1
  Multimeter4/1 -> [V3]
  [rho] -> Gain4/1
  Gain1/1 -> Sum3/2
  [V3] -> Mux4/1
  [Vref3] -> Sum3/1
  [y3] -> Gain1/1
  [It3] -> Mux4/2
  Gain4/1 -> Sum2/1, Scope7/1
  Integrator/1 -> Mux4/3
  Sum3/1 -> Integrator/1
  Sum2/1 -> To Workspace1/1, [y3]
  Mux4/1 -> To Workspace/1, [x3]
  [x3] -> Sum2/2
  [Il3] -> Mux1/1
  Mux1/1 -> State-Space1/1
  [secondary] -> Product/2
  Current Measurement/1 -> [Inet3]
  Product/1 -> Mux1/4
  [Inet3] -> Product/1
  [Vref3] -> Mux1/2
  [Vt3d] -> Mux1/3
  State-Space1/1 -> [xavg3]
  connections:
  Ground1/LConn1 -- Voltage Measurement/LConn2
  IGBT1/RConn1 -- AC Current Source/RConn1 -- Capacitance/RConn1 -- Ground/LConn1 -- DC Voltage Source/LConn1 -- Diode1/LConn1
  Capacitance/LConn1 -- Current Measurement/LConn1 -- AC Current Source/LConn1 -- Inductance/RConn1
  IGBT/LConn1 -- Diode/RConn1 -- DC Voltage Source/RConn1
  Resistance/RConn1 -- Inductance/LConn1
  IGBT/RConn1 -- Resistance/LConn1 -- Voltage Measurement/LConn1 -- Diode1/RConn1 -- IGBT1/LConn1 -- Diode/LConn1
  Current Measurement/RConn1 -- PCC3/RConn1

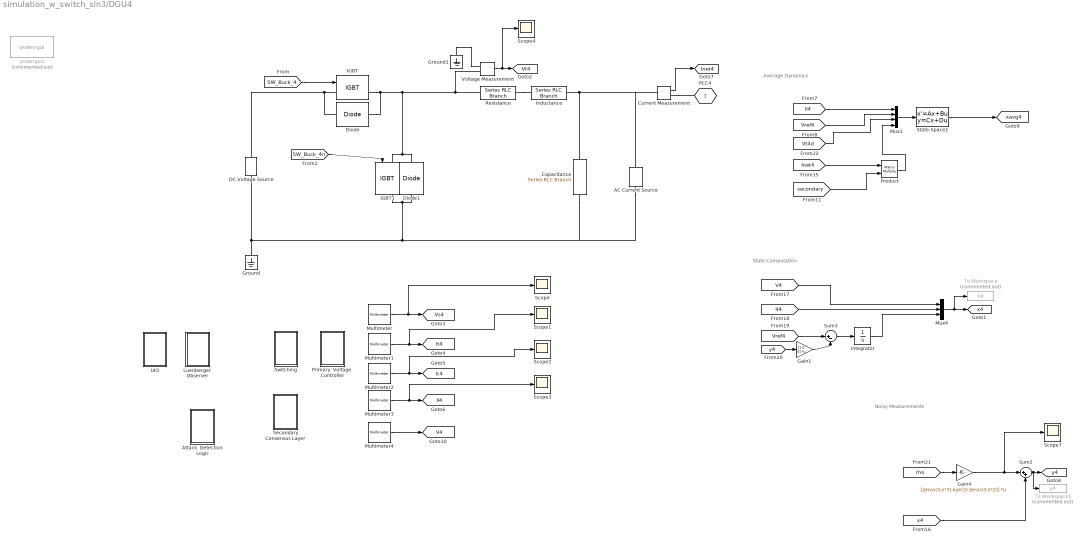
== system simulation_w_switch_sln3/DGU4 ==
  note: Noisy Measurements
  note: State Computation
  note: Average Dynamics
  AC Current Source : powerlib/Electrical Sources/AC Current Source  Amplitude=13  Phase=90  Frequency=0  SampleTime=0  Measurements=Current
      settings: SourceProductBaseCode=PS
  Attack  Detection Logic : Subsystem
  Capacitance : powerlib/Elements/Series RLC Branch  LConnTagsString=__new0  RConnTagsString=__new0  BranchType=C  Resistance=1  Inductance=1.8e-3  SetiL0=off  InitialCurrent=0  Capacitance=DGU(4).Ct  Setx0=off  InitialVoltage=48  Measurements=Branch voltage and current
  Current Measurement : powerlib/Measurements/Current Measurement  PhasorSimulation=off  OutputType=Magnitude  PSBequivalent=0
  DC Voltage Source : powerlib/Electrical Sources/DC Voltage Source  Amplitude=Vs  Measurements=Voltage
  Diode : powerlib/Power Electronics/Diode  Ron=0.001  Lon=0  Vf=0.8  IC=0  UseSnubber=0  Rs=500  Cs=250e-9  Measurements=off
  Diode1 : powerlib/Power Electronics/Diode  Ron=0.001  Lon=0  Vf=0.8  IC=0  UseSnubber=0  Rs=500  Cs=250e-9  Measurements=off
  Gain1 : Gain  Gain=[1 0 0]  Multiplication=Matrix(K*u) (u vector)
  Gain4 : Gain  Gain=[zeros(3,n*3) eye(3) zeros(3,n*2)]  Multiplication=Matrix(K*u) (u vector)
  Ground : powerlib/Elements/Ground  LConnTagsString=a
  Ground1 : powerlib/Elements/Ground  LConnTagsString=a
  IGBT : powerlib/Power Electronics/IGBT  Ron=0.001  Lon=0  Vf=1  Tf=1e-6  Tt=2e-6  IC=0  Rs=1e5  Cs=inf  Measurements=on
  IGBT1 : powerlib/Power Electronics/IGBT  Ron=0.001  Lon=0  Vf=1  Tf=1e-6  Tt=2e-6  IC=0  Rs=1e5  Cs=inf  Measurements=on
  Inductance : powerlib/Elements/Series RLC Branch  LConnTagsString=__new0  RConnTagsString=__new0  BranchType=L  Resistance=1  Inductance=DGU(4).Lt  SetiL0=off  InitialCurrent=13  Capacitance=1e-6  Setx0=off  InitialVoltage=0  Measurements=None
  Integrator : Integrator
  Luenberger  Observer : Subsystem
  Multimeter : powerlib/Measurements/Multimeter  PhasorSimulation=off  OutputType=Complex  sel=10  L=30  Gain=1  yselected={'Usrc: DGU4/DC Voltage Source'};  PSBOutputType=1  PSBequivalent=0  AxesSetting=[0,0.1,-100,100]  Display=0  SavedBlockNames=-11
  Multimeter1 : powerlib/Measurements/Multimeter  PhasorSimulation=off  OutputType=Complex  sel=16  L=30  Gain=1  yselected={'Ib: DGU4/Resistance'};  PSBOutputType=1  PSBequivalent=0  AxesSetting=[0,0.1,-100,100]  Display=0  SavedBlockNames=-11
  Multimeter2 : powerlib/Measurements/Multimeter  PhasorSimulation=off  OutputType=Complex  sel=15  L=30  Gain=1  yselected={'Ib: DGU4/Capacitance'};  PSBOutputType=1  PSBequivalent=0  AxesSetting=[0,0.1,-100,100]  Display=0  SavedBlockNames=-11
  Multimeter3 : powerlib/Measurements/Multimeter  PhasorSimulation=off  OutputType=Complex  sel=28  L=30  Gain=1  yselected={'Isrc: DGU4/AC Current Source'};  PSBOutputType=1  PSBequivalent=0  AxesSetting=[0,0.1,-100,100]  Display=0  SavedBlockNames=-11
  Multimeter4 : powerlib/Measurements/Multimeter  PhasorSimulation=off  OutputType=Complex  sel=2  L=30  Gain=1  yselected={'Ub: DGU4/Capacitance'};  PSBOutputType=1  PSBequivalent=0  AxesSetting=[0,0.1,-100,100]  Display=0  SavedBlockNames=-11
  Mux1 : Mux
  Mux4 : Mux  Inputs=3
  Primary  Voltage  Controller : Subsystem
  Product : Product  Multiplication=Matrix(*)
  Resistance : powerlib/Elements/Series RLC Branch  LConnTagsString=__new0  RConnTagsString=__new0  BranchType=R  Resistance=DGU(4).Rt  Inductance=1e-3  SetiL0=off  InitialCurrent=0  Capacitance=1e-6  Setx0=off  InitialVoltage=0  Measurements=Branch current
  Scope{,1..4,7} (6 alike) : Scope
  Secondary Consensus Layer : Subsystem
  State-Space1 : StateSpace  A=DGU(4).Aii  B=[DGU(4).M DGU(4).B [-1/DGU(4).Ct;0;0]]  C=eye(3)  D=zeros(n,4)  InitialCondition=0
  Sum2 : Sum  Inputs=|++
  Sum3 : Sum  Inputs=|+-
  Switching : Subsystem
  To Workspace : ToWorkspace  Commented=on  VariableName=x4  SaveFormat=Timeseries  SampleTime=tSampData
  To Workspace1 : ToWorkspace  Commented=on  VariableName=y4  SaveFormat=Timeseries  SampleTime=tSampData
  UIO : Subsystem
  Voltage Measurement : powerlib/Measurements/Voltage Measurement  PhasorSimulation=off  OutputType=Complex  PSBequivalent=0
  powergui1 : powerlib/powergui  Priority=1  Commented=on  SimulationMode=Continuous  SampleTime=50e-6  frequency=60  Iterations=50  frequencyindice=60  Pbase=100e6  ErrMax=1e-4  UnitsV=kV  UnitsW=MW  buscounter=0  FunctionMessages=off  echomessages=off  EnableUseOfTLC=off  CurrentSourceSwitches=off  DisableSnubberDevices=off  DisableRonSwitches=off  DisableVfSwitches=off  DisplayEquations=off  AutomaticDiscreteSolvers=off  SolverType=Tustin/Backward Euler (TBE)  Interpol=off  ExternalGateDelay=off  methode=off  Ts=100  x0status=blocks  SPID=on  SwTol=0  HookPort=off  NonlinearTolerance=1e-4  nMaxIteration=100  ContinueOnMaxIteration=off  RestoreLinks=warning  ResistiveCurrentMeasurement=off  Frange=[0:2:500]  Ylog=off  Xlog=on  ShowGrid=off  save=off  variable=ZData  structure=0  ZoomFFT=off  StartTime=0.0  cycles=1  DisplayStyle=1  fundamental=60  FreqAxis=off  MaxFrequency=1000  frequencyindicesteady=1  RmsSteady=1  display=off
  PCC4 : PMIOPort  Tag=PMCPort  Side=Left
  tag scope: Ic4=global, Il4=global, Inet4=global, It4=global, V4=global, Vs4=global, Vt4=global, x4=global, xavg4=global, y4=global
  wires:
  Multimeter/1 -> Scope/1, [Vs4]
  Multimeter2/1 -> Scope2/1, [Ic4]
  Voltage Measurement/1 -> Scope4/1, [Vt4]
  Multimeter1/1 -> Scope1/1, [It4]
  [SW_Buck_4n] -> IGBT1/1
  Multimeter3/1 -> Scope3/1, [Il4]
  [SW_Buck_4] -> IGBT/1
  Multimeter4/1 -> [V4]
  [rho] -> Gain4/1
  Gain1/1 -> Sum3/2
  [V4] -> Mux4/1
  [Vref4] -> Sum3/1
  [y4] -> Gain1/1
  [It4] -> Mux4/2
  Gain4/1 -> Sum2/1, Scope7/1
  Integrator/1 -> Mux4/3
  Sum3/1 -> Integrator/1
  Sum2/1 -> To Workspace1/1, [y4]
  Mux4/1 -> To Workspace/1, [x4]
  [x4] -> Sum2/2
  [Il4] -> Mux1/1
  Mux1/1 -> State-Space1/1
  [secondary] -> Product/2
  Current Measurement/1 -> [Inet4]
  Product/1 -> Mux1/4
  [Inet4] -> Product/1
  [Vref4] -> Mux1/2
  [Vt4d] -> Mux1/3
  State-Space1/1 -> [xavg4]
  connections:
  Ground1/LConn1 -- Voltage Measurement/LConn2
  IGBT1/RConn1 -- AC Current Source/RConn1 -- Capacitance/RConn1 -- Ground/LConn1 -- DC Voltage Source/LConn1 -- Diode1/LConn1
  Capacitance/LConn1 -- Current Measurement/LConn1 -- AC Current Source/LConn1 -- Inductance/RConn1
  IGBT/LConn1 -- Diode/RConn1 -- DC Voltage Source/RConn1
  Resistance/RConn1 -- Inductance/LConn1
  IGBT/RConn1 -- Resistance/LConn1 -- Voltage Measurement/LConn1 -- Diode1/RConn1 -- IGBT1/LConn1 -- Diode/LConn1
  Current Measurement/RConn1 -- PCC4/RConn1
